simulink model "Problem_4"  (R2020a)
settings: Solver=VariableStepAuto  StartTime=0.0  StopTime=10.0  RelTol=1e-3
PreLoadFcn:
  | L = 2.75E-6;
  | R = 4;
  | b = 3.5077E-6;
  | J = 3.2284E-6;
  | K = 0.0274;
undefined symbols (not defined in the file or in its folder): Kd, Ki, Kp
settings Model: DataDictionary=Dictionary_Problem4.sldd  Creator=Admin  LastModifiedBy=Admin

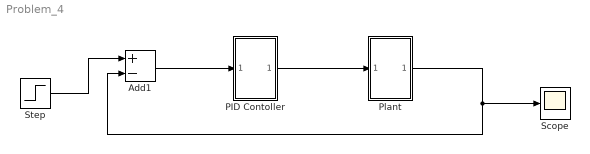
== system Problem_4 ==
  Add1 : Sum  Inputs=+-
  PID Contoller : Subsystem
  Plant : Subsystem
  Scope : Scope
  Step : Step  Time=0  After=500  SampleTime=0
  wires:
  Plant/1(Out1) -> Scope/1, Add1/2
  Step/1 -> Add1/1
  Add1/1 -> PID Contoller/1(In1)
  PID Contoller/1(Out1) -> Plant/1(In1)

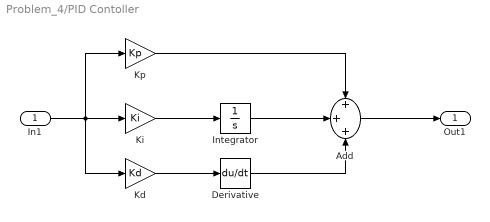
== system Problem_4/PID Contoller ==
  In1 : Inport
  Add : Sum  Inputs=+++
  Derivative : Derivative
  Integrator : Integrator
  Kd : Gain  Gain=Kd
  Ki : Gain  Gain=Ki
  Kp : Gain  Gain=Kp
  Out1 : Outport
  wires:
  Ki/1 -> Integrator/1
  Derivative/1 -> Add/3
  In1/1 -> Kp/1, Kd/1, Ki/1
  Add/1 -> Out1/1
  Kp/1 -> Add/1
  Integrator/1 -> Add/2
  Kd/1 -> Derivative/1

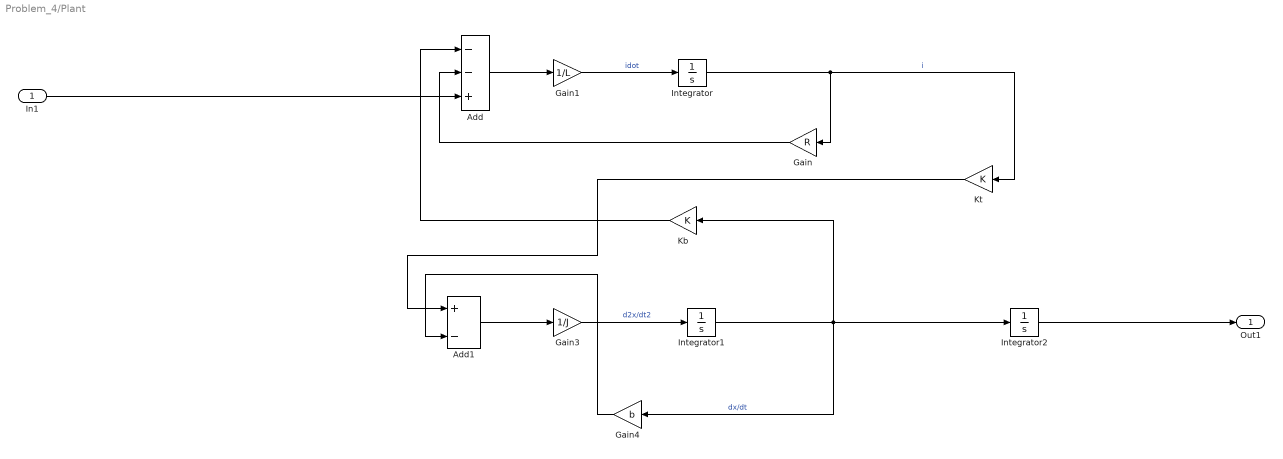
== system Problem_4/Plant ==
  In1 : Inport
  Add : Sum  Inputs=--+
  Add1 : Sum  Inputs=+-
  Gain : Gain  Gain=R
  Gain1 : Gain  Gain=1/L
  Gain3 : Gain  Gain=1/J
  Gain4 : Gain  Gain=b
  Integrator : Integrator
  Integrator1 : Integrator
  Integrator2 : Integrator
  Kb : Gain  Gain=K
  Kt : Gain  Gain=K
  Out1 : Outport
  wires:
  Add1/1 -> Gain3/1
  Gain1/1 -> Integrator/1  "idot"
  Add/1 -> Gain1/1
  Integrator1/1 -> Integrator2/1, Kb/1, Gain4/1  "dx/dt"
  Gain3/1 -> Integrator1/1  "d2x/dt2"
  Kb/1 -> Add/1
  Gain4/1 -> Add1/2
  Kt/1 -> Add1/1
  Gain/1 -> Add/2
  Integrator/1 -> Gain/1, Kt/1  "i"
  Integrator2/1 -> Out1/1
  In1/1 -> Add/3
